simulink model "pid_sim"  (R2016b)
settings: Solver=VariableStepAuto  StartTime=0.0  StopTime=10.0  RelTol=1e-3
settings Model: Creator=Han Wei  LastModifiedBy=Han Wei

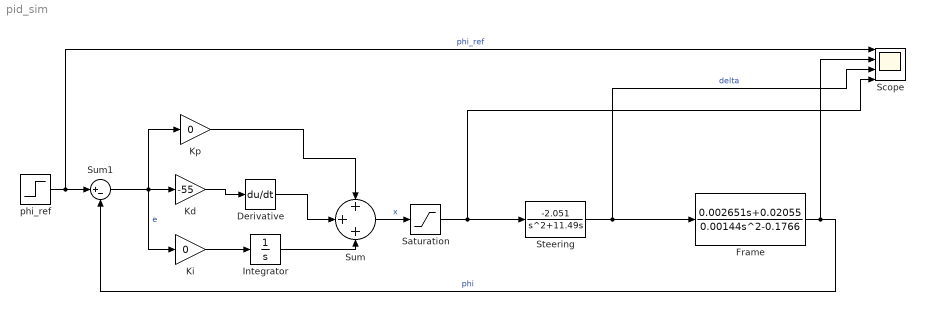
== system pid_sim ==
  Derivative : Derivative
  Frame : TransferFcn  Numerator=[0.002651 0.02055]  Denominator=[0.00144 0 -0.1766]
  Integrator : Integrator
  Kd : Gain  Gain=-55
  Ki : Gain  Gain=0
  Kp : Gain  Gain=0
  Saturation : Saturate  UpperLimit=100  LowerLimit=-100
  Scope : Scope  NumInputPorts=4
  Steering : TransferFcn  Numerator=[-2.051]  Denominator=[1 11.49 0]
  Sum : Sum  Inputs=3
  Sum1 : Sum  Inputs=|+-
  phi_ref : Step  After=0.3  SampleTime=0
  wires:
  Kp/1 -> Sum/1
  Derivative/1 -> Sum/2
  Integrator/1 -> Sum/3
  Kd/1 -> Derivative/1
  Ki/1 -> Integrator/1
  Sum/1 -> Saturation/1  "x"
  Steering/1 -> Scope/3, Frame/1  "delta"
  Frame/1 -> Sum1/2, Scope/2  "phi"
  Sum1/1 -> Ki/1, Kp/1, Kd/1  "e"
  phi_ref/1 -> Scope/1, Sum1/1  "phi_ref"
  Saturation/1 -> Steering/1, Scope/4
